simulink model "Modelo5_1_2_C_1_zero"  (R2020a)
settings: Solver=VariableStepAuto  StartTime=0.0  StopTime=10.0  RelTol=1e-3
values from neighbouring files (symbols this model uses):
  b_eq = b_m + b_l/(r^2)    (= 2.19444444444e-05)    [LTI_vs_LPV_vs_NL_realimentado.m]    (also in Modelo_linealizado.m)
  J_eq = J_m + J_l/(r^2)    (= 1.97847222222e-05)    [LTI_vs_LPV_vs_NL_realimentado.m]    (also in Modelo_linealizado.m)
  L_q = 5.8/1000    (= 0.0058)    [Curvas_carc.m]    (also in LTI_vs_LPV_vs_NL_realimentado.m; Modelo_linealizado.m)
  lambda_m = 0.01546    [Curvas_carc.m]    (also in LTI_vs_LPV_vs_NL_realimentado.m = 0.016; Modelo_linealizado.m = 0.016)
  Pp = 3    [AnalisisDeEstabilidad.m]    (also in LTI_vs_LPV_vs_NL_realimentado.m; Modelo_linealizado.m; parametros.m)
  r = 120    [AnalisisDeEstabilidad.m]    (also in LTI_vs_LPV_vs_NL_realimentado.m; Modelo_linealizado.m; parametros.m)
  R_s = 1.02    [Curvas_carc.m]    (also in LTI_vs_LPV_vs_NL_realimentado.m = R_s_o; Modelo_linealizado.m = 0.348)
  z = -60    [Modelo_linealizado.m]
settings Model: Creator=Juan  LastModifiedBy=Juan

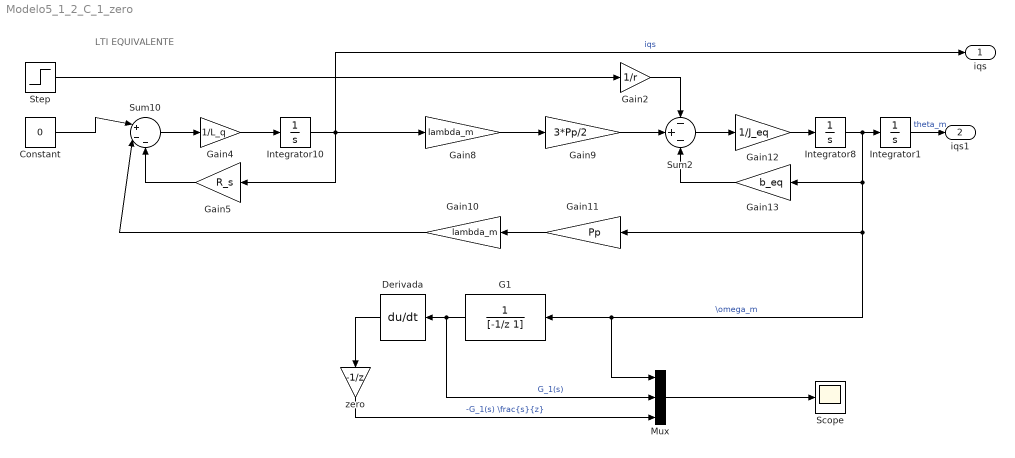
== system Modelo5_1_2_C_1_zero ==
  note: LTI EQUIVALENTE
  Constant : Constant  Value=0
  Derivada : Derivative
  G1 : TransferFcn  Denominator=[-1/z 1]
      settings: AttributesFormatString=%<Tag>
  Gain10 : Gain  Gain=lambda_m
  Gain11 : Gain  Gain=Pp
  Gain12 : Gain  Gain=1/J_eq
  Gain13 : Gain  Gain=b_eq
  Gain2 : Gain  Gain=1/r
  Gain4 : Gain  Gain=1/L_q
  Gain5 : Gain  Gain=R_s
  Gain8 : Gain  Gain=lambda_m
  Gain9 : Gain  Gain=3*Pp/2
  Integrator1 : Integrator
  Integrator10 : Integrator
  Integrator8 : Integrator
  Mux : Mux  Inputs=3
  Scope : Scope
  Step : Step  After=6.28  SampleTime=0
  Sum10 : Sum  Inputs=|+--
  Sum2 : Sum  Inputs=-+-
  zero : Gain  Gain=-1/z
  iqs : Outport
  iqs1 : Outport  Port=2
  wires:
  Mux/1 -> Scope/1
  Integrator1/1 -> iqs1/1  "theta_m"
  Sum10/1 -> Gain4/1
  Gain11/1 -> Gain10/1
  Gain10/1 -> Sum10/2
  Sum2/1 -> Gain12/1
  Derivada/1 -> zero/1
  G1/1 -> Mux/2, Derivada/1  "G_1(s)"
  Integrator10/1 -> iqs/1, Gain8/1, Gain5/1  "iqs"
  Gain13/1 -> Sum2/3
  Gain12/1 -> Integrator8/1
  Constant/1 -> Sum10/1
  Gain8/1 -> Gain9/1
  Integrator8/1 -> Mux/1, G1/1, Gain11/1, Gain13/1, Integrator1/1  "\\omega_m"
  Gain4/1 -> Integrator10/1
  zero/1 -> Mux/3  "-G_1(s) \\frac{s}{z}"
  Step/1 -> Gain2/1
  Gain5/1 -> Sum10/3
  Gain9/1 -> Sum2/2
  Gain2/1 -> Sum2/1
